simulink model "subsystem_depth_metric"  (R2020a)
settings: Solver=VariableStepAuto  StartTime=0.0  StopTime=10.0  RelTol=1e-3
settings Model: Creator=00081598  LastModifiedBy=00081598

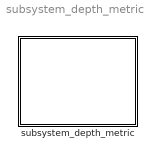
== system subsystem_depth_metric ==
  subsystem_depth_metric : Subsystem

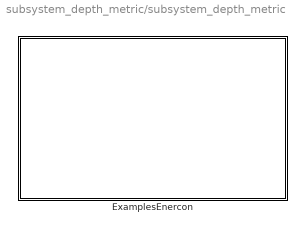
== system subsystem_depth_metric/subsystem_depth_metric ==
  ExamplesEnercon : Subsystem

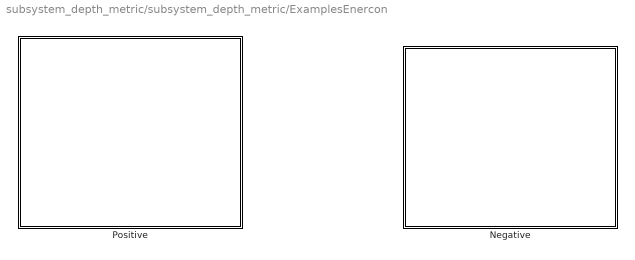
== system subsystem_depth_metric/subsystem_depth_metric/ExamplesEnercon ==
  Negative : Subsystem
  Positive : Subsystem

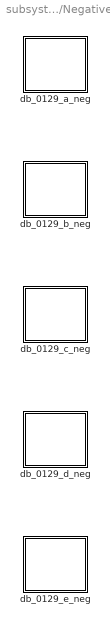
== system subsystem_depth_metric/subsystem_depth_metric/ExamplesEnercon/Negative ==
  db_0129_a_neg : Stateflow chart  TreatAsAtomicUnit=on
  db_0129_b_neg : Stateflow chart  TreatAsAtomicUnit=on
  db_0129_c_neg : Stateflow chart  TreatAsAtomicUnit=on
  db_0129_d_neg : Stateflow chart  TreatAsAtomicUnit=on
  db_0129_e_neg : Stateflow chart  TreatAsAtomicUnit=on

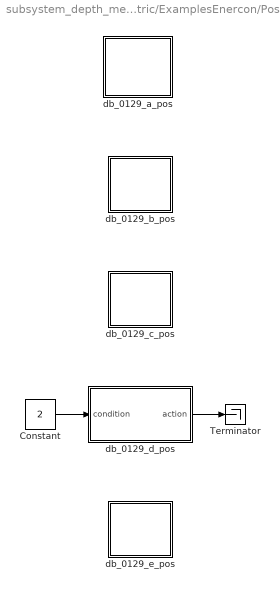
== system subsystem_depth_metric/subsystem_depth_metric/ExamplesEnercon/Positive ==
  Constant : Constant  Value=2
  Terminator : Terminator
  db_0129_a_pos : Stateflow chart  TreatAsAtomicUnit=on
  db_0129_b_pos : Stateflow chart  TreatAsAtomicUnit=on
  db_0129_c_pos : Stateflow chart  TreatAsAtomicUnit=on
  db_0129_d_pos : Stateflow chart  TreatAsAtomicUnit=on
  db_0129_e_pos : Stateflow chart  TreatAsAtomicUnit=on
  wires:
  db_0129_d_pos/1(action) -> Terminator/1
  Constant/1 -> db_0129_d_pos/1(condition)

== stateflow chart subsystem_depth_metric/ExamplesEnercon/Negative/db_0129_b_neg ==
  state StateA
  state StateB
  (default) -> StateA
  StateA -> StateB
  StateB -> StateA

== stateflow chart subsystem_depth_metric/ExamplesEnercon/Positive/db_0129_c_pos ==
  state State001
  state State002
  state State003
  (default) -> State001
  State002 -> State003
  State001 -> State002
  State003 -> State001

== stateflow chart subsystem_depth_metric/ExamplesEnercon/Negative/db_0129_c_neg ==
  state StateABC
  state StateBBC
  state StateCBA
  (default) -> StateABC
  StateABC -> StateBBC
  StateBBC -> StateCBA
  StateCBA -> StateABC

== stateflow chart subsystem_depth_metric/ExamplesEnercon/Positive/db_0129_d_pos ==
  state State0005 [parallel]
    settings: executionOrder=1
    state State0001
    state State0002
    (default) -> State0001
    State0001 -> State0002 [order 1] : [condition > 0]
    State0002 -> State0001 : [condition > 1]
    State0001 -> (junction 35) [order 2] : [condition == 3]
  state State0007 [parallel]
    settings: executionOrder=2
    state State0003
    state State0004
    (default) -> State0003
    State0003 -> State0004 [order 1] : [condition > 0]
    State0004 -> State0003 : [condition > 1]
    State0003 -> (junction 43) [order 2] : [condition == 3]
  state State0008 [parallel]
    settings: executionOrder=3
    (default) -> (junction 12)
    (junction 12) -> (junction 13) [order 1] : [condition > 0]
    (junction 13) -> (junction 14) : {
        | action = 1;
        | }
    (junction 14) -> (junction 12)
    (junction 12) -> (junction 15) [order 2] : {
        | action = 2;
        | }
  state State0006 [parallel]
    settings: executionOrder=4
    (default) -> (junction 21)
    (junction 21) -> (junction 22) [order 1] : [condition > 0]
    (junction 21) -> (junction 26) [order 2]
    (junction 22) -> (junction 24) : {
        | action = 2;
        | }
    (junction 24) -> (junction 26)
    (junction 26) -> (junction 28) : {
        | action = 1;
        | }
  data: action output; condition input

== stateflow chart subsystem_depth_metric/ExamplesEnercon/Negative/db_0129_d_neg ==
  state StatesS
  state StateFF
  state StateSB
    (default) -> (junction 8)
    (junction 8) -> (junction 9)
    (junction 10) -> (junction 9)
  (default) -> StatesS
  StatesS -> StateSB
  StateFF -> StatesS
  StateSB -> StateFF

== stateflow chart subsystem_depth_metric/ExamplesEnercon/Positive/db_0129_e_pos ==
  state State004 [parallel]
    settings: executionOrder=1
    (default) -> (junction 2)
    (junction 2) -> (junction 25) [order 1]
    (junction 25) -> (junction 3) [order 1]
    (junction 25) -> (junction 29) [order 2]
    (junction 2) -> (junction 27) [order 2]
    (junction 3) -> (junction 5)
    (junction 29) -> (junction 27)
    (junction 27) -> (junction 4)
    (junction 5) -> (junction 4)
    (junction 4) -> (junction 6)
  state State005 [parallel]
    settings: executionOrder=2
    (default) -> (junction 14)
    (junction 14) -> (junction 15) [order 1]
    (junction 14) -> (junction 16) [order 2]
    (junction 15) -> (junction 17)
    (junction 17) -> (junction 16)
    (junction 16) -> (junction 18)

== stateflow chart subsystem_depth_metric/ExamplesEnercon/Negative/db_0129_e_neg ==
  state StateE1
    (default) -> (junction 3)
    (junction 3) -> (junction 4) [order 1]
    (junction 4) -> (junction 6) [order 1]
    (junction 3) -> (junction 17) [order 2]
    (junction 4) -> (junction 19) [order 2]
    (junction 6) -> (junction 8)
    (junction 19) -> (junction 17)
    (junction 17) -> (junction 10)
    (junction 22) -> (junction 10)
    (junction 8) -> (junction 22)
    (junction 10) -> (junction 15)
  (default) -> StateE1

== stateflow chart subsystem_depth_metric/ExamplesEnercon/Negative/db_0129_a_neg ==
  state State0004 [parallel]
    settings: executionOrder=2
    (default) -> (junction 20)
    (junction 20) -> (junction 23) [order 2]
    (junction 25) -> (junction 23) [order 1]
    (junction 20) -> (junction 21) [order 1]
    (junction 23) -> (junction 29)
    (junction 25) -> (junction 27) [order 2]
    (junction 27) -> (junction 21)
    (junction 21) -> (junction 32)
    (junction 29) -> (junction 32)
    (junction 32) -> (junction 35)
  state State0003 [parallel]
    settings: executionOrder=1
    state ABCC
    state ABCD
    state ABCE
    (default) -> ABCC
    ABCC -> ABCD [order 1]
    ABCD -> ABCC
    ABCC -> ABCE [order 2]

== stateflow chart subsystem_depth_metric/ExamplesEnercon/Positive/db_0129_b_pos ==
  state State0001
  state State0002
  (default) -> State0001
  State0001 -> State0002
  State0002 -> State0001

== stateflow chart subsystem_depth_metric/ExamplesEnercon/Positive/db_0129_a_pos ==
  state State003 [parallel]
    settings: executionOrder=1
    state State001
    state State002
    (default) -> State001
    State001 -> State002 [order 1]
    State002 -> State001
    State001 -> (junction 12) [order 2]
  state State004 [parallel]
    settings: executionOrder=2
    (default) -> (junction 19)
    (junction 19) -> (junction 20) [order 1]
    (junction 19) -> (junction 24) [order 2]
    (junction 20) -> (junction 21)
    (junction 21) -> (junction 24)
    (junction 24) -> (junction 27)
